simulink model "TRNG_test10"  (R2020a)
settings: Solver=VariableStepAuto  StartTime=0.0  StopTime=10.0  RelTol=1e-3
undefined symbols (not defined in the file): AXI4, Lite
libraries: xbsIndex_r4 x27
settings Model: Creator=ringl  LastModifiedBy=ringl

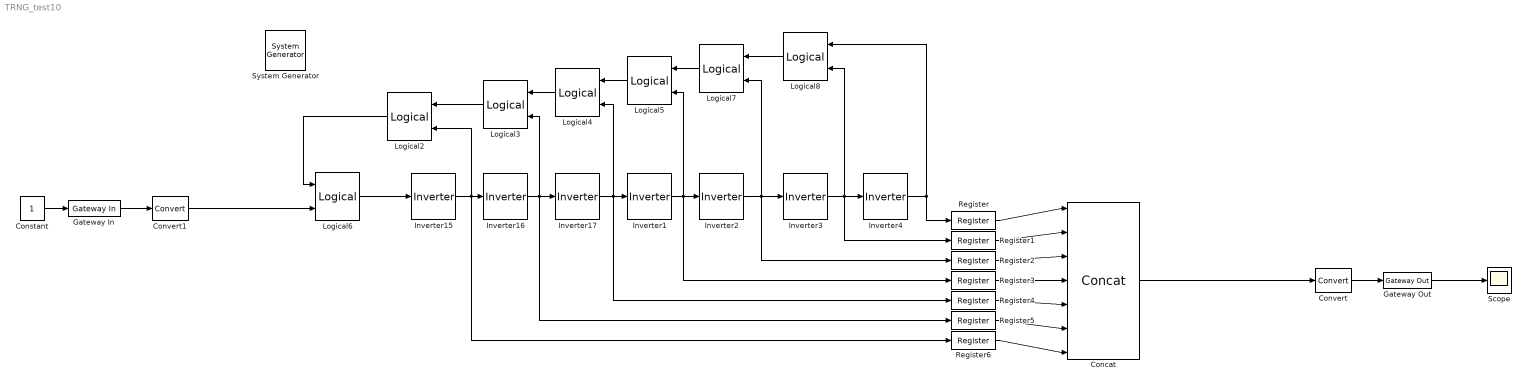
== system TRNG_test10 ==
  " System Generator" : xbsIndex_r4/ System Generator  Tag=genX  xilinxfamily=zynq  part=xc7z020  speed=-1  package=clg400  synthesis_tool=Vivado  clock_wrapper=Clock Enables  directory=./netlist  proj_type=Vivado  Synth_file=Vivado Synthesis Defaults  Impl_file=Vivado Implementation Defaults  testbench=off  simulink_period=1  sysclk_period=10  dcm_input_clock_period=10  incr_netlist=off  trim_vbits=Everywhere in SubSystem  dbl_ovrd=According to Block Masks  core_generation=According to Block Masks  run_coregen=off  deprecated_control=off  eval_field=0  block_type=sysgen
  Concat : xbsIndex_r4/Concat  num_inputs=7  dbl_ovrd=off  block_type=concat
  Constant : Constant
  Convert : xbsIndex_r4/Convert  gui_display_data_type=Fixed-point  arith_type="Signed  (2's comp)"  n_bits=32  bin_pt=0  float_type=Single  exp_bits=8  fraction_bits=24  quantization=Truncate  overflow=Wrap  en=off  latency=1  pipeline=off  dbl_ovrd=off  block_type=convert
  Convert1 : xbsIndex_r4/Convert  gui_display_data_type=Fixed-point  arith_type=Unsigned  n_bits=1  bin_pt=0  float_type=Single  exp_bits=8  fraction_bits=24  quantization=Truncate  overflow=Wrap  en=off  latency=1  pipeline=off  dbl_ovrd=off  block_type=convert
  Gateway In : xbsIndex_r4/Gateway In  gui_display_data_type=Fixed-point  arith_type="Signed  (2's comp)"  n_bits=32  bin_pt=0  preci_type=Single  exp_width=8  frac_width=24  rows=1  columns=1  quantization="Round  (unbiased: +/- Inf)"  overflow=Saturate  period=1  UseAsADC=off  ADCChannel='1'  interface=AXI4-Lite  automatic_assignment=on  address_offset=hex2dec('00')  intf_name=''  intf_description=''  default_value=0  timing_constraint=None  locs_specified=off  LOCs={}  io_standard={}  inherit_from_input=off  hdl_port=on  dbl_ovrd=off  block_type=gatewayin
  Gateway Out : xbsIndex_r4/Gateway Out  inherit_from_input=off  hdl_port=on  rows=1  columns=1  UseAsDAC=off  DACChannel='1'  interface=AXI4-Lite  automatic_assignment=on  address_offset=hex2dec('00')  intf_name=''  intf_description=''  timing_constraint=None  locs_specified=off  LOCs={}  io_standard={}  block_type=gatewayout
  Inverter{1..4,15..17} (7 alike) : xbsIndex_r4/Inverter  en=off  latency=1  dbl_ovrd=off  block_type=inv
  Logical{2..5,7..8} (6 alike) : xbsIndex_r4/Logical  logical_function=XOR  inputs=2  en=off  latency=1  precision=Full  arith_type=Unsigned  n_bits=16  bin_pt=0  align_bp=on  dbl_ovrd=off  block_type=logical
  Logical6 : xbsIndex_r4/Logical  logical_function=AND  inputs=2  en=off  latency=1  precision=User Defined  arith_type=Unsigned  n_bits=1  bin_pt=0  align_bp=on  dbl_ovrd=off  block_type=logical
  Register{,1..6} (7 alike) : xbsIndex_r4/Register  init=0  rst=off  en=off  dbl_ovrd=off  block_type=register
  Scope : Scope
  wires:
  Gateway Out/1 -> Scope/1
  Convert/1 -> Gateway Out/1
  Concat/1 -> Convert/1
  Gateway In/1 -> Convert1/1
  Constant/1 -> Gateway In/1
  Inverter15/1 -> Register6/1, Logical2/2, Inverter16/1
  Logical6/1 -> Inverter15/1
  Logical2/1 -> Logical6/1
  Inverter16/1 -> Register5/1, Logical3/2, Inverter17/1
  Inverter17/1 -> Logical4/2, Register4/1, Inverter1/1
  Inverter1/1 -> Register3/1, Logical5/2, Inverter2/1
  Inverter2/1 -> Register2/1, Logical7/2, Inverter3/1
  Inverter3/1 -> Register1/1, Logical8/2, Inverter4/1
  Convert1/1 -> Logical6/2
  Logical3/1 -> Logical2/1
  Logical4/1 -> Logical3/1
  Logical5/1 -> Logical4/1
  Logical7/1 -> Logical5/1
  Logical8/1 -> Logical7/1
  Inverter4/1 -> Register/1, Logical8/1
  Register/1 -> Concat/1
  Register1/1 -> Concat/2
  Register2/1 -> Concat/3
  Register3/1 -> Concat/4
  Register4/1 -> Concat/5
  Register5/1 -> Concat/6
  Register6/1 -> Concat/7
